simulink model "heat_exchanger_test01_sim"  (R2017b)
settings: Solver=VariableStepAuto  StartTime=0.0  StopTime=0  RelTol=1e-3
values from neighbouring files (symbols this model uses):
  c = conversion_factors()    [heat_exchanger_test01.m]    (also in reactor_test_ideal_gas_models_comparison.m)
undefined symbols (not defined in the file or in its folder): CoolProp
libraries: thermochemical x14
settings Model: Creator=fferrucc  LastModifiedBy=fferrucc

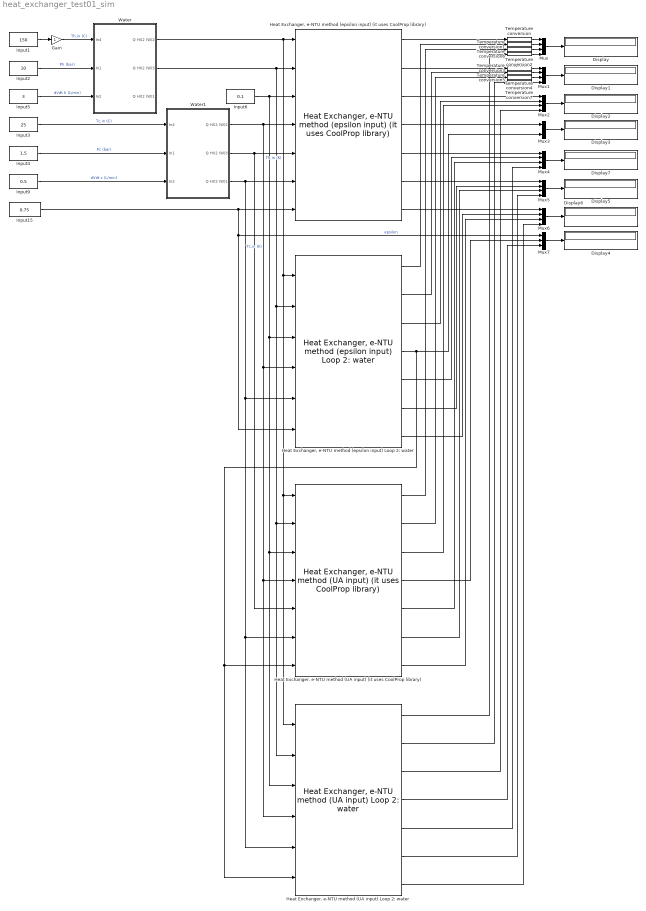
== system heat_exchanger_test01_sim ==
  Display{,1..7} (8 alike) : Display
  Gain : Gain
  "Heat Exchanger, e-NTU method (UA input) (it uses CoolProp library)" : thermochemical/Heat exchangers/Heat Exchanger, e-NTU method (UA input) (it uses CoolProp library)  fluidName_1=Ammonia  fluidName_2=Water  flowType=Cross-flow, Cmin mixed, Cmax unmixed
      settings: SourceProductName=@ Thermochemical
  "Heat Exchanger, e-NTU method (UA input) Loop 2: water" : thermochemical/Heat exchangers/Heat Exchanger, e-NTU method (UA input) Loop 2: water  fluid=fluid  flowType=Cross-flow, Cmin mixed, Cmax unmixed  cp_water_J_K_mol=75.3260
      settings: SourceProductName=@ Thermochemical
  "Heat Exchanger, e-NTU method (epsilon input) (it uses CoolProp library)" : thermochemical/Heat exchangers/Heat Exchanger, e-NTU method (epsilon input) (it uses CoolProp library)  fluidName_1=Ammonia  fluidName_2=Water  flowType=Cross-flow, Cmin mixed, Cmax unmixed
      settings: SourceProductName=@ Thermochemical
  "Heat Exchanger, e-NTU method (epsilon input) Loop 2: water" : thermochemical/Heat exchangers/Heat Exchanger, e-NTU method (epsilon input) Loop 2: water  fluid=fluid  flowType=Cross-flow, Cmin mixed, Cmax unmixed  cp_water_J_K_mol=75.3260
      settings: SourceProductName=@ Thermochemical
  Input1 : Constant  Value=150
  Input15 : Constant  Value=0.75
  Input2 : Constant  Value=10
  Input3 : Constant  Value=25
  Input4 : Constant  Value=1.5
  Input5 : Constant  Value=3
  Input6 : Constant  Value=0.1
  Input9 : Constant  Value=0.5
  Mux{,1..2,4..6} (6 alike) : Mux
  Mux3 : Mux  Inputs=2
  Mux7 : Mux  Inputs=3
  Temperature conversion{,1..7} (8 alike) : thermochemical/Conversions/Temperature conversion  sel=K --> °C
      settings: SourceProductName=@ Thermochemical
  Water : Subsystem
  Water1 : Subsystem
  wires:
  Input3/1 -> Water1/1(In4)  "Tc,in (C)"
  Input4/1 -> Water1/2(In1)  "Pc (bar)"
  Input9/1 -> Water1/3(In2)  "dVdt c (L/min)"
  Input15/1 -> "Heat Exchanger, e-NTU method (epsilon input) (it uses CoolProp library)"/7, Mux7/1, "Heat Exchanger, e-NTU method (epsilon input) Loop 2: water"/6  "epsilon"
  Water1/3(Q HX2 (W)1) -> "Heat Exchanger, e-NTU method (epsilon input) Loop 2: water"/5, "Heat Exchanger, e-NTU method (UA input) Loop 2: water"/5, "Heat Exchanger, e-NTU method (UA input) (it uses CoolProp library)"/6, "Heat Exchanger, e-NTU method (epsilon input) (it uses CoolProp library)"/6
  Water1/1(Q HX2 (W)2) -> "Heat Exchanger, e-NTU method (UA input) Loop 2: water"/4, "Heat Exchanger, e-NTU method (UA input) (it uses CoolProp library)"/4, "Heat Exchanger, e-NTU method (epsilon input) Loop 2: water"/4, "Heat Exchanger, e-NTU method (epsilon input) (it uses CoolProp library)"/4  "Tc,in (K)"
  Water/1(Q HX2 (W)2) -> "Heat Exchanger, e-NTU method (epsilon input) Loop 2: water"/1, "Heat Exchanger, e-NTU method (UA input) Loop 2: water"/1, "Heat Exchanger, e-NTU method (UA input) (it uses CoolProp library)"/1, "Heat Exchanger, e-NTU method (epsilon input) (it uses CoolProp library)"/1  "Th,in (K)"
  Input6/1 -> "Heat Exchanger, e-NTU method (UA input) Loop 2: water"/3, "Heat Exchanger, e-NTU method (UA input) (it uses CoolProp library)"/3, "Heat Exchanger, e-NTU method (epsilon input) Loop 2: water"/3, "Heat Exchanger, e-NTU method (epsilon input) (it uses CoolProp library)"/3
  Input5/1 -> Water/3(In2)  "dVdt h (L/min)"
  Water/2(Q HX2 (W)3) -> "Heat Exchanger, e-NTU method (UA input) (it uses CoolProp library)"/2, "Heat Exchanger, e-NTU method (UA input) Loop 2: water"/2, "Heat Exchanger, e-NTU method (epsilon input) Loop 2: water"/2, "Heat Exchanger, e-NTU method (epsilon input) (it uses CoolProp library)"/2
  Input2/1 -> Water/2(In1)  "Ph (bar)"
  Gain/1 -> Water/1(In4)  "Th,in (C)"
  Water1/2(Q HX2 (W)3) -> "Heat Exchanger, e-NTU method (UA input) (it uses CoolProp library)"/5, "Heat Exchanger, e-NTU method (epsilon input) (it uses CoolProp library)"/5
  "Heat Exchanger, e-NTU method (epsilon input) Loop 2: water"/4 -> "Heat Exchanger, e-NTU method (UA input) (it uses CoolProp library)"/7, "Heat Exchanger, e-NTU method (UA input) Loop 2: water"/6, Mux3/2
  "Heat Exchanger, e-NTU method (epsilon input) (it uses CoolProp library)"/1 -> Temperature conversion/1
  "Heat Exchanger, e-NTU method (epsilon input) Loop 2: water"/1 -> Temperature conversion1/1
  Mux/1 -> Display/1
  "Heat Exchanger, e-NTU method (UA input) (it uses CoolProp library)"/1 -> Temperature conversion2/1
  Mux1/1 -> Display1/1
  "Heat Exchanger, e-NTU method (epsilon input) (it uses CoolProp library)"/2 -> Temperature conversion3/1
  "Heat Exchanger, e-NTU method (epsilon input) Loop 2: water"/2 -> Temperature conversion4/1
  "Heat Exchanger, e-NTU method (UA input) (it uses CoolProp library)"/2 -> Temperature conversion5/1
  Mux2/1 -> Display2/1
  "Heat Exchanger, e-NTU method (epsilon input) (it uses CoolProp library)"/3 -> Mux2/1
  "Heat Exchanger, e-NTU method (epsilon input) (it uses CoolProp library)"/4 -> Mux3/1
  "Heat Exchanger, e-NTU method (epsilon input) Loop 2: water"/3 -> Mux2/2
  "Heat Exchanger, e-NTU method (UA input) (it uses CoolProp library)"/3 -> Mux2/3
  "Heat Exchanger, e-NTU method (epsilon input) (it uses CoolProp library)"/5 -> Mux4/1
  "Heat Exchanger, e-NTU method (epsilon input) Loop 2: water"/5 -> Mux4/2
  Mux5/1 -> Display5/1
  "Heat Exchanger, e-NTU method (epsilon input) (it uses CoolProp library)"/6 -> Mux5/1
  "Heat Exchanger, e-NTU method (epsilon input) Loop 2: water"/6 -> Mux5/2
  "Heat Exchanger, e-NTU method (UA input) (it uses CoolProp library)"/6 -> Mux5/3
  Mux6/1 -> Display6/1
  "Heat Exchanger, e-NTU method (epsilon input) (it uses CoolProp library)"/7 -> Mux6/1
  "Heat Exchanger, e-NTU method (epsilon input) Loop 2: water"/7 -> Mux6/2
  "Heat Exchanger, e-NTU method (UA input) (it uses CoolProp library)"/7 -> Mux6/3
  Mux7/1 -> Display4/1
  "Heat Exchanger, e-NTU method (UA input) (it uses CoolProp library)"/4 -> Mux7/2
  "Heat Exchanger, e-NTU method (UA input) (it uses CoolProp library)"/5 -> Mux4/3
  Temperature conversion/1 -> Mux/1
  Temperature conversion1/1 -> Mux/2
  Temperature conversion2/1 -> Mux/3
  Temperature conversion3/1 -> Mux1/1
  Temperature conversion4/1 -> Mux1/2
  Temperature conversion5/1 -> Mux1/3
  Input1/1 -> Gain/1
  Mux3/1 -> Display3/1
  Mux4/1 -> Display7/1
  Temperature conversion6/1 -> Mux/4
  Temperature conversion7/1 -> Mux1/4
  "Heat Exchanger, e-NTU method (UA input) Loop 2: water"/1 -> Temperature conversion6/1
  "Heat Exchanger, e-NTU method (UA input) Loop 2: water"/2 -> Temperature conversion7/1
  "Heat Exchanger, e-NTU method (UA input) Loop 2: water"/5 -> Mux4/4
  "Heat Exchanger, e-NTU method (UA input) Loop 2: water"/6 -> Mux5/4
  "Heat Exchanger, e-NTU method (UA input) Loop 2: water"/7 -> Mux6/4
  "Heat Exchanger, e-NTU method (UA input) Loop 2: water"/3 -> Mux2/4
  "Heat Exchanger, e-NTU method (UA input) Loop 2: water"/4 -> Mux7/3

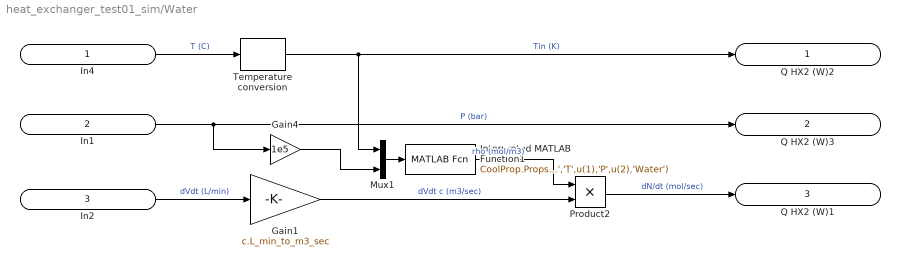
== system heat_exchanger_test01_sim/Water ==
  In4 : Inport
  In1 : Inport  Port=2
  In2 : Inport  Port=3
  Gain1 : Gain  Gain=c.L_min_to_m3_sec
  Gain4 : Gain  Gain=1e5
  Interpreted MATLAB Function1 : MATLABFcn  MATLABFcn=CoolProp.PropsSI('DMOLAR','T',u(1),'P',u(2),'Water')  OutputDimensions=1
  Mux1 : Mux  Inputs=2
  Product2 : Product
  Temperature conversion : thermochemical/Conversions/Temperature conversion  sel=°C --> K
      settings: SourceProductName=@ Thermochemical
  Q HX2 (W)2 : Outport
  Q HX2 (W)3 : Outport  Port=2
  Q HX2 (W)1 : Outport  Port=3
  wires:
  In1/1 -> Q HX2 (W)3/1, Gain4/1  "P (bar)"
  Gain1/1 -> Product2/2  "dVdt c (m3/sec)"
  In4/1 -> Temperature conversion/1  "T (C)"
  In2/1 -> Gain1/1  "dVdt (L/min)"
  Product2/1 -> Q HX2 (W)1/1  "dN/dt (mol/sec)"
  Gain4/1 -> Mux1/2
  Temperature conversion/1 -> Mux1/1, Q HX2 (W)2/1  "Tin (K)"
  Interpreted MATLAB Function1/1 -> Product2/1  "rho (mol/m3)"
  Mux1/1 -> Interpreted MATLAB Function1/1

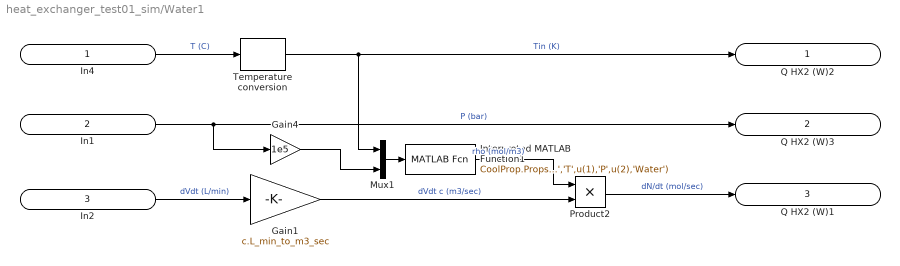
== system heat_exchanger_test01_sim/Water1 ==
  In4 : Inport
  In1 : Inport  Port=2
  In2 : Inport  Port=3
  Gain1 : Gain  Gain=c.L_min_to_m3_sec
  Gain4 : Gain  Gain=1e5
  Interpreted MATLAB Function1 : MATLABFcn  MATLABFcn=CoolProp.PropsSI('DMOLAR','T',u(1),'P',u(2),'Water')  OutputDimensions=1
  Mux1 : Mux  Inputs=2
  Product2 : Product
  Temperature conversion : thermochemical/Conversions/Temperature conversion  sel=°C --> K
      settings: SourceProductName=@ Thermochemical
  Q HX2 (W)2 : Outport
  Q HX2 (W)3 : Outport  Port=2
  Q HX2 (W)1 : Outport  Port=3
  wires:
  Mux1/1 -> Interpreted MATLAB Function1/1
  Interpreted MATLAB Function1/1 -> Product2/1  "rho (mol/m3)"
  Temperature conversion/1 -> Q HX2 (W)2/1, Mux1/1  "Tin (K)"
  Gain4/1 -> Mux1/2
  Product2/1 -> Q HX2 (W)1/1  "dN/dt (mol/sec)"
  In2/1 -> Gain1/1  "dVdt (L/min)"
  In4/1 -> Temperature conversion/1  "T (C)"
  Gain1/1 -> Product2/2  "dVdt c (m3/sec)"
  In1/1 -> Gain4/1, Q HX2 (W)3/1  "P (bar)"
